simulink model "ObjectImaging"  (Simulink 4.00)
settings: Solver=ode45  StartTime=0.0  StopTime=10.0  RelTol=1e-3
values from neighbouring files (symbols this model uses):
  c = camera(1000,1000,256,256,512,512)    [initHBVS.m]    (also in pose0.mat = ; pose1.mat = ; sim1.mat = ; task_endeff.mat = )
  p = reshape(u,2,n)    [CamView.m]    (also in initHBVS.m = polyhedra([0.0 0.0 0; 0.25 0.25 0; -0.25 0.25 0; -0.25 -0.25; pose0.mat = ; pose1.mat = ; sim1.mat = )
  T0c_0 = T0c    [initHBVS.m]    (also in sim1.mat = )
  T0o =     [pose0.mat]    (also in pose1.mat; sim1.mat; task_endeff.mat; task_stereo.mat)
undefined symbols (not defined in the file or in its folder): coords, get, GetHMatrix
libraries: vs x6
settings Model: LastModifiedBy=quique

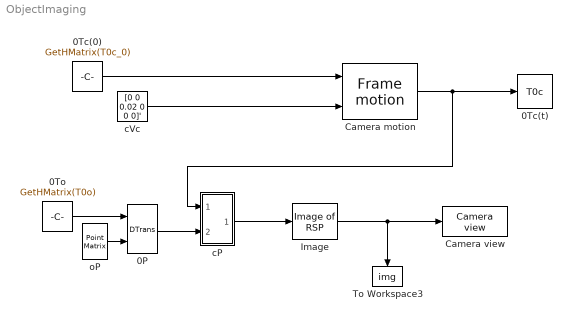
== system ObjectImaging ==
  0P : vs/Features/DTrans
      settings: RTWFcnNameOpts=Auto  RTWFileNameOpts=Auto
  0Tc(0) : Constant  Value=GetHMatrix(T0c_0)  VectorParams1D=off
  0Tc(t) : ToWorkspace  VariableName=T0c  SampleTime=-1  SaveFormat=StructureWithTime
  0To : Constant  Value=GetHMatrix(T0o)  VectorParams1D=off
  Camera motion : vs/Pose/Frame motion
      settings: RTWFcnNameOpts=Auto  RTWFileNameOpts=Auto
  Camera view : vs/Camera/Camera view  ms=15  em=normal  umin=0  umax=get(c,'hres')-1  vmin=0  vmax=get(c,'vres')-1  st=-1
  Image : vs/Camera/Image of RSP  fu=get(c,'fu')  fv=get(c,'fv')  u0=get(c,'u0')  v0=get(c,'v0')
  To Workspace3 : ToWorkspace  VariableName=img  SampleTime=-1  SaveFormat=StructureWithTime
      settings: Orientation=down
  cP : Subsystem  AncestorBlock=vs/Features/ITrans
      settings: RTWFcnNameOpts=Auto  RTWFileNameOpts=Auto
  cVc : Constant  Value=[0 0 0.02 0 0 0]'  VectorParams1D=off
  oP : vs/Features/Point Matrix  m=coords(p)
  wires:
  0Tc(0)/1 -> Camera motion/1
  Camera motion/1 -> 0Tc(t)/1, cP/1(aTb)
  cVc/1 -> Camera motion/2
  cP/1(bP) -> Image/1
  Image/1 -> Camera view/1, To Workspace3/1
  0P/1 -> cP/2(aP)
  oP/1 -> 0P/2
  0To/1 -> 0P/1

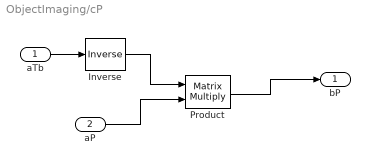
== system ObjectImaging/cP ==
  aTb : Inport  Port=1  LatchInput=off
  aP : Inport  Port=2  LatchInput=off
  Inverse : vs/Pose/Inverse
      settings: RTWFcnNameOpts=Auto  RTWFileNameOpts=Auto
  Product : Product  Inputs=2  Multiplication=Matrix(*)  SaturateOnIntegerOverflow=on
  bP : Outport  Port=1
  wires:
  Inverse/1 -> Product/1
  aTb/1 -> Inverse/1
  Product/1 -> bP/1
  aP/1 -> Product/2
